simulink model "CurrentComp_v21"  (R2013a)
settings: Solver=ode45  StartTime=0.0  StopTime=10.0  MaxStep=1e-4  RelTol=1e-3
InitFcn:
  | param=evalin('base','param;');
  | 
  | JR=str2num(param.JR);
  | KMT=str2num(param.KMT);
  | Rc=str2num(param.Rc);
  | Lc=str2num(param.Lc);
  | KFR=str2num(param.KFR);
  | KTB=str2num(param.KTB);
  | KBM=str2num(param.KBM);
  | Rsh=str2num(param.Rsh);
StartFcn:
  | sprintf('Info (%s):\nKTB = %.1e\nKBM = %.1e\n', gcs, KTB, KBM)
model workspace (MATLAB code in the model file):
  | %param=evalin('base','loadGalvoParam(4);');
  | param=evalin('base','param;');
  | 
  | JR=str2num(param.JR);
  | KMT=str2num(param.KMT);
  | Rc=str2num(param.Rc);
  | Lc=str2num(param.Lc);
  | KFR=str2num(param.KFR);
  | KTB=str2num(param.KTB);
  | KBM=str2num(param.KBM);
  | Rsh=str2num(param.Rsh);
libraries: simulink x1
settings Model: BufferReuse=off  Creator=mainster  LastModifiedBy=mainster
settings DataIOCC: SaveOutput=off  SaveTime=off
settings OptimizationCC: InlineParams=on  BufferReuse=off
settings DebuggingCC: InitInArrayFormatMsg=none
settings ModelReferenceCC: ModelReferenceMinAlgLoopOccurrences=on

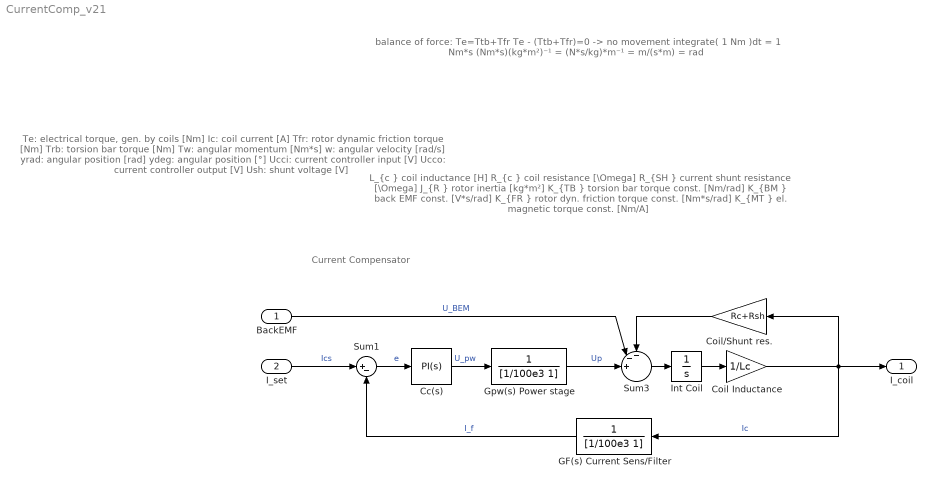
== system CurrentComp_v21 ==
  note: Current Compensator
  note: Te: 		electrical torque, gen. by coils		[Nm]
      |  Ic: 			coil current							[A]
      |  Tfr:		rotor dynamic friction torque 		[Nm]
      |  Trb:		torsion bar torque					[Nm]
      |  Tw:		angular momentum				[Nm*s]
      |  w:			angular velocity 					[rad/s]
      |  yrad:		angular position 					[rad]
      |  ydeg:		angular position 					[°]
      |  Ucci:		current controller input				[V]
      |  Ucco:		current controller output			[V]
      |  Ush:		shunt voltage						[V]
  note: L_{c  }	coil inductance 							[H]
      |  R_{c  }	coil resistance							[\Omega]
      |  R_{SH }	current shunt resistance				[\Omega]
      |  J_{R  }	rotor inertia 							[kg*m²]
      |  K_{TB }	torsion bar torque const. 			[Nm/rad]
      |  K_{BM }	back EMF const.							[V*s/rad]
      |  K_{FR }	rotor dyn. friction torque const.	[Nm*s/rad]
      |  K_{MT }	el. magnetic torque const.			[Nm/A]
  note: balance of force: 	Te=Ttb+Tfr
      | 					Te - (Ttb+Tfr)=0  ->  no movement
      |
      |  integrate( 1 Nm )dt = 1 Nm*s
      |  (Nm*s)(kg*m²)⁻¹ = (N*s/kg)*m⁻¹ = m/(s*m) = rad
  BackEMF : Inport
  I_set : Inport  Port=2
  Cc(s) : simulink/Continuous/PID Controller  Controller=PI  TimeDomain=Continuous-time  SampleTime=1  IntegratorMethod=Forward Euler  FilterMethod=Forward Euler  Form=Ideal  P=2.58986900309333  I=14540.01765706  D=0  N=100  InitialConditionSource=internal  InitialConditionForIntegrator=0  InitialConditionForFilter=0  ExternalReset=none  LimitOutput=off  UpperSaturationLimit=inf  LowerSaturationLimit=-inf  LinearizeAsGain=on  AntiWindupMode=none  Kb=1  TrackingMode=off  Kt=1  PParamMin=[]  PParamMax=[]  IParamMin=[]  IParamMax=[]  DParamMin=[]  DParamMax=[]  NParamMin=[]  NParamMax=[]  KbParamMin=[]  KbParamMax=[]  KtParamMin=[]  KtParamMax=[]  POutMin=[]  POutMax=[]  IOutMin=[]  IOutMax=[]  DOutMin=[]  DOutMax=[]  NOutMin=[]  NOutMax=[]  KbOutMin=[]  KbOutMax=[]  KtOutMin=[]  KtOutMax=[]  IntegratorOutMin=[]  IntegratorOutMax=[]  FilterOutMin=[]  FilterOutMax=[]  SumOutMin=[]  SumOutMax=[]  SumI1OutMin=[]  SumI1OutMax=[]  SumI2OutMin=[]  SumI2OutMax=[]  SumI3OutMin=[]  SumI3OutMax=[]  SumDOutMin=[]  SumDOutMax=[]  SaturationOutMin=[]  SaturationOutMax=[]  IntegratorContinuousStateAttributes=''  IntegratorStateMustResolveToSignalObject=off  IntegratorRTWStateStorageClass=Auto  FilterContinuousStateAttributes=''  FilterStateMustResolveToSignalObject=off  FilterRTWStateStorageClass=Auto
  Coil Inductance : Gain  Gain=1/Lc
  Coil/Shunt res. : Gain  Gain=Rc+Rsh
  GF(s) Current Sens/Filter : TransferFcn  Denominator=[1/100e3 1]
  Gpw(s) Power stage : TransferFcn  Denominator=[1/100e3 1]
  Int Coil : Integrator
  Sum1 : Sum  Inputs=|+-
  Sum3 : Sum  Inputs=--+||
  I_coil : Outport
  wires:
  I_set/1 -> Sum1/1  "Ics"
  Sum1/1 -> Cc(s)/1  "e"
  Coil Inductance/1 -> I_coil/1, GF(s) Current Sens/Filter/1, Coil/Shunt res./1  "Ic"
  Coil/Shunt res./1 -> Sum3/1
  Sum3/1 -> Int Coil/1
  Int Coil/1 -> Coil Inductance/1
  Cc(s)/1 -> Gpw(s) Power stage/1  "U_pw"
  Gpw(s) Power stage/1 -> Sum3/3  "Up"
  BackEMF/1 -> Sum3/2  "U_BEM"
  GF(s) Current Sens/Filter/1 -> Sum1/2  "I_f"
